simulink model "redocking_site"  (R2020b)
settings: Solver=FixedStepDiscrete  StartTime=0.0  StopTime=stopTime  FixedStep=2.0833333333333333e-05  RelTol=1e-3
values from neighbouring files (symbols this model uses):
  t_rd_init = t_rd_rest + 0.02e-3*spont - t_rd_jump    (= 0.0156)    [modelparameters.m]
  unitRateInterval = -log(randNums(k))/tdres    [SpikeGenerator_matt.m]    (also in modelparameters.m = 87745)
libraries: hdlsllib x1
settings Model: Creator=Ross  LastModifiedBy=tyler
settings SolverCC: AutoInsertRateTranBlk=on
settings DataIOCC: SaveOutput=off  SaveTime=off  ReturnWorkspaceOutputs=off
settings OptimizationCC: BlockReduction=off  ConditionallyExecuteInputs=off  DefaultParameterBehavior=Inlined
settings DebuggingCC: ReadBeforeWriteMsg=DisableAll  WriteAfterWriteMsg=DisableAll  WriteAfterReadMsg=DisableAll  AlgebraicLoopMsg=error  MultiTaskDSMMsg=none  SingleTaskRateTransMsg=error  PregeneratedLibrarySubsystemCodeDiagnostic=none  ArithmeticOperatorsInVariantConditions=warning
settings HardwareCC: ProdBitPerPointer=32  ProdBitPerSizeT=32  ProdBitPerPtrDiffT=32  ProdLargestAtomicFloat=None  ProdIntDivRoundTo=Undefined  ProdEndianess=Unspecified  ProdWordSize=32  ProdHWDeviceType=ASIC/FPGA->ASIC/FPGA  TargetBitPerPointer=64  TargetBitPerSizeT=64  TargetBitPerPtrDiffT=64  TargetLongLongMode=on  TargetIntDivRoundTo=Zero  TargetEndianess=LittleEndian  TargetWordSize=64  TargetHWDeviceType=Custom Processor->MATLAB Host Computer  ProdEqTarget=off
settings ModelReferenceCC: UpdateModelReferenceTargets=IfOutOfDate
settings SFSimCC: SFSimEcho=off  SimUseLocalCustomCode=off  CustomCodeUndefinedFunction=UseInterfaceOnly
settings RTWCC: RTWUseLocalCustomCode=off

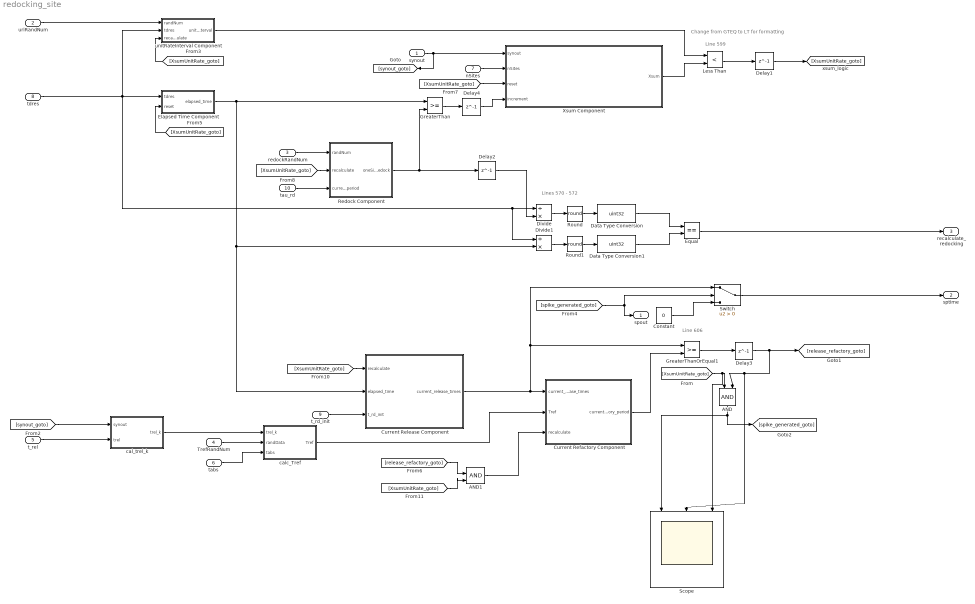
== system redocking_site ==
  note: Change from GTEQ to LT for formatting
  note: Line 606
  note: Lines 570 - 572
  note: Line 599
  synout : Inport  OutDataTypeStr=single  PortDimensions=1  SampleTime=[2.0833333333333333e-05,0]
  uriRandNum : Inport  Port=2  OutDataTypeStr=single  PortDimensions=1  SampleTime=[2.0833333333333333e-05,0]
  redockRandNum : Inport  Port=3  OutDataTypeStr=single  PortDimensions=1  SampleTime=[2.0833333333333333e-05,0]
  TrefRandNum : Inport  Port=4  OutDataTypeStr=single  PortDimensions=1  SampleTime=[2.0833333333333333e-05,0]
  t_rel : Inport  Port=5  OutDataTypeStr=single  PortDimensions=1  SampleTime=[2.0833333333333333e-05,0]
  tabs : Inport  Port=6  OutDataTypeStr=single  PortDimensions=1  SampleTime=[2.0833333333333333e-05,0]
  nSites : Inport  Port=7  OutDataTypeStr=single  PortDimensions=1  SampleTime=[2.0833333333333333e-05,0]
  tdres : Inport  Port=8  OutDataTypeStr=single  PortDimensions=1  SampleTime=[2.0833333333333333e-05,0]
  t_rd_init : Inport  Port=9  OutDataTypeStr=single  PortDimensions=1  SampleTime=[2.0833333333333333e-05,0]
  tau_rd : Inport  Port=10  OutDataTypeStr=single  PortDimensions=1  SampleTime=[2.0833333333333333e-05,0]
  AND : Logic  IconShape=distinctive  AllPortsSameDT=off  OutDataTypeStr=boolean
  AND1 : Logic  IconShape=distinctive  AllPortsSameDT=off  OutDataTypeStr=boolean
  Constant : Constant  Value=0  OutDataTypeStr=single  SampleTime=-1
  Current Refactory Component : Subsystem
  Current Release Component : Subsystem
  Data Type Conversion : DataTypeConversion  OutDataTypeStr=uint32
  Data Type Conversion1 : DataTypeConversion  OutDataTypeStr=uint32
  Delay{1..4} (4 alike) : Delay  DelayLength=1
  Divide : Product  Inputs=/*
  Divide1 : Product  Inputs=/*
  Elapsed Time Component : Subsystem
  Equal : RelationalOperator  Operator===  OutDataTypeStr=boolean  RndMeth=Simplest
  GreaterThan : RelationalOperator  OutDataTypeStr=boolean  RndMeth=Simplest
  GreaterThanOrEqual1 : RelationalOperator  OutDataTypeStr=boolean  RndMeth=Simplest
  Less Than : RelationalOperator  Operator=<  OutDataTypeStr=boolean  RndMeth=Simplest
  Redock Component : Subsystem
  Round : Rounding  Operator=round
  Round1 : Rounding  Operator=round
  Scope : Scope  NumInputPorts=3
  Switch : Switch  Criteria=u2 > Threshold
  Xsum Component : Subsystem
  cal_trel_k : Subsystem
  calc_Tref : Subsystem
  unitRateInterval Component : Subsystem
  spout : Outport  OutDataTypeStr=boolean  PortDimensions=1  SampleTime=[2.0833333333333333e-05,0]  InitialOutput=0
  sptime : Outport  Port=2  OutDataTypeStr=single  PortDimensions=1  SampleTime=[2.0833333333333333e-05,0]  InitialOutput=0
  recalculate_redocking : Outport  Port=3  OutDataTypeStr=boolean  PortDimensions=1  SampleTime=[2.0833333333333333e-05,0]
  wires:
  [spike_generated_goto] -> spout/1, Switch/2
  GreaterThanOrEqual1/1 -> Delay3/1
  Constant/1 -> Switch/3
  unitRateInterval Component/1(unitRateInterval) -> Less Than/1
  Xsum Component/1(Xsum) -> Less Than/2
  redockRandNum/1 -> Redock Component/1(randNum)
  [XsumUnitRate_goto] -> AND1/2
  [XsumUnitRate_goto] -> Elapsed Time Component/2(reset)
  [XsumUnitRate_goto] -> Xsum Component/3(reset)
  [XsumUnitRate_goto] -> unitRateInterval Component/3(recalculate)
  Delay2/1 -> Divide/2
  [XsumUnitRate_goto] -> Current Release Component/1(recalculate)
  calc_Tref/1(Tref) -> Current Refactory Component/2(Tref)
  [synout_goto] -> cal_trel_k/1(synout)
  uriRandNum/1 -> unitRateInterval Component/1(randNum)
  Delay1/1 -> [XsumUnitRate_goto]
  cal_trel_k/1(trel_k) -> calc_Tref/1(trel_k)
  t_rel/1 -> cal_trel_k/2(trel)
  Switch/1 -> sptime/1
  Equal/1 -> recalculate_redocking/1
  tabs/1 -> calc_Tref/3(tabs)
  Delay3/1 -> AND/2, Scope/2, [release_refactory_goto]
  Less Than/1 -> Delay1/1
  tdres/1 -> Divide1/1, Divide/1, unitRateInterval Component/2(tdres), Elapsed Time Component/1(tdres)
  Divide1/1 -> Round1/1
  [release_refactory_goto] -> AND1/1
  nSites/1 -> Xsum Component/2(nSites)
  [XsumUnitRate_goto] -> Redock Component/2(recalculate)
  Data Type Conversion1/1 -> Equal/2
  t_rd_init/1 -> Current Release Component/3(t_rd_init)
  TrefRandNum/1 -> calc_Tref/2(randData)
  Round/1 -> Data Type Conversion/1
  Round1/1 -> Data Type Conversion1/1
  tau_rd/1 -> Redock Component/3(current_redocking_period)
  synout/1 -> Xsum Component/1(synout), [synout_goto]
  AND/1 -> [spike_generated_goto], Scope/1
  [XsumUnitRate_goto] -> Scope/3, AND/1
  AND1/1 -> Current Refactory Component/3(recalculate)
  Divide/1 -> Round/1
  Data Type Conversion/1 -> Equal/1
  Current Refactory Component/1(current_refactory_period) -> GreaterThanOrEqual1/2
  Current Release Component/1(current_release_times) -> GreaterThanOrEqual1/1, Switch/1, Current Refactory Component/1(current_release_times)
  Elapsed Time Component/1(elapsed_time) -> GreaterThan/1, Current Release Component/2(elapsed_time), Divide1/2
  GreaterThan/1 -> Delay4/1
  Delay4/1 -> Xsum Component/4(increment)
  Redock Component/1(oneSiteRedock) -> GreaterThan/2, Delay2/1

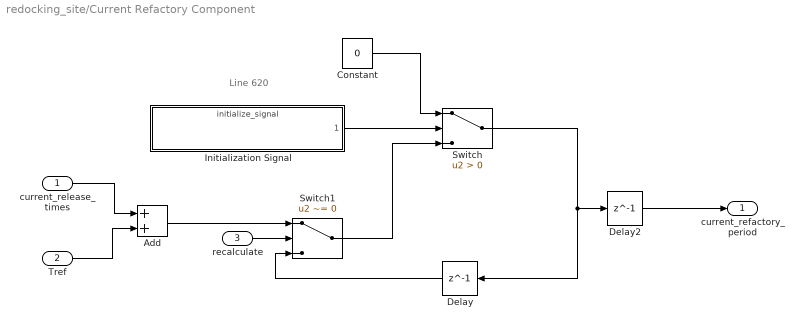
== system redocking_site/Current Refactory Component ==
  note: Line 620
  current_release_times : Inport
  Tref : Inport  Port=2
  recalculate : Inport  Port=3
  Add : Sum
  Constant : Constant  Value=0  OutDataTypeStr=single  SampleTime=-1
  Delay : Delay  DelayLength=1
  Delay2 : Delay  DelayLength=1
  Initialization Signal : ModelReference  ModelNameDialog=initialize_signal  SimulationMode=Normal  ModelReferenceVersion=1.282
  Switch : Switch  Criteria=u2 > Threshold  OutDataTypeStr=single
  Switch1 : Switch  Criteria=u2 ~= 0  OutDataTypeStr=single
  current_refactory_period : Outport
  wires:
  Delay/1 -> Switch1/3
  Switch/1 -> Delay2/1, Delay/1
  Switch1/1 -> Switch/3
  current_release_times/1 -> Add/1
  Tref/1 -> Add/2
  recalculate/1 -> Switch1/2
  Initialization Signal/1 -> Switch/2
  Constant/1 -> Switch/1
  Add/1 -> Switch1/1
  Delay2/1 -> current_refactory_period/1

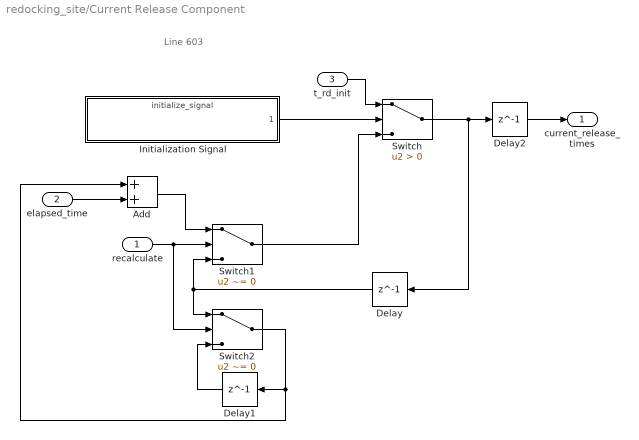
== system redocking_site/Current Release Component ==
  note: Line 603
  recalculate : Inport
  elapsed_time : Inport  Port=2
  t_rd_init : Inport  Port=3
  Add : Sum
  Delay : Delay  DelayLength=1
  Delay1 : Delay  DelayLength=1
  Delay2 : Delay  DelayLength=1
  Initialization Signal : ModelReference  ModelNameDialog=initialize_signal  SimulationMode=Normal  ModelReferenceVersion=1.282
  Switch : Switch  Criteria=u2 > Threshold  OutDataTypeStr=single
  Switch1 : Switch  Criteria=u2 ~= 0  OutDataTypeStr=single
  Switch2 : Switch  Criteria=u2 ~= 0  OutDataTypeStr=single
  current_release_times : Outport
  wires:
  Delay/1 -> Switch2/1, Switch1/3
  Switch/1 -> Delay2/1, Delay/1
  Switch1/1 -> Switch/3
  recalculate/1 -> Switch2/2, Switch1/2
  Add/1 -> Switch1/1
  Switch2/1 -> Add/1, Delay1/1
  elapsed_time/1 -> Add/2
  Initialization Signal/1 -> Switch/2
  t_rd_init/1 -> Switch/1
  Delay1/1 -> Switch2/3
  Delay2/1 -> current_release_times/1

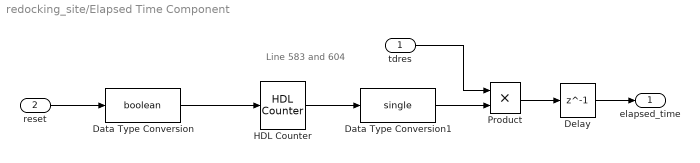
== system redocking_site/Elapsed Time Component ==
  note: Line 583 and 604
  tdres : Inport
  reset : Inport  Port=2
  Data Type Conversion : DataTypeConversion  OutDataTypeStr=boolean
  Data Type Conversion1 : DataTypeConversion  OutDataTypeStr=single
  Delay : Delay  DelayLength=1
  HDL Counter : hdlsllib/Sources/HDL Counter  CountType=Count limited  CountInit=0  CountStep=1  CountMax=1023  CountFromType=Initial value  CountFrom=0  CountResetPort=on  CountLoadPort=off  CountEnbPort=off  CountDirPort=off  CountDataType=Unsigned  CountWordLen=10  CountFracLen=0  CountSampTime=-1
  Product : Product  OutDataTypeStr=single
  elapsed_time : Outport
  wires:
  Data Type Conversion1/1 -> Product/2
  Data Type Conversion/1 -> HDL Counter/1
  Product/1 -> Delay/1
  tdres/1 -> Product/1
  HDL Counter/1 -> Data Type Conversion1/1
  reset/1 -> Data Type Conversion/1
  Delay/1 -> elapsed_time/1

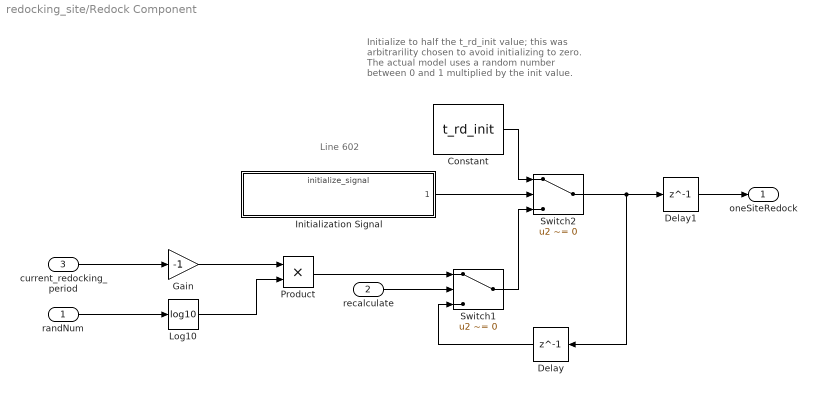
== system redocking_site/Redock Component ==
  note: Line 602
  note: Initialize to half the t_rd_init value; this was
      | arbitrarility chosen to avoid initializing to zero.
      | The actual model uses a random number
      | between 0 and 1 multiplied by the init value.
  randNum : Inport
  recalculate : Inport  Port=2
  current_redocking_period : Inport  Port=3
  Constant : Constant  Value=t_rd_init  OutDataTypeStr=single  SampleTime=-1
  Delay : Delay  DelayLength=1
  Delay1 : Delay  DelayLength=1
  Gain : Gain  Gain=-1
  Initialization Signal : ModelReference  ModelNameDialog=initialize_signal  SimulationMode=Normal  ModelReferenceVersion=1.282
  Log10 : Math  Operator=log10  SaturateOnIntegerOverflow=on
  Product : Product
  Switch1 : Switch  Criteria=u2 ~= 0  OutDataTypeStr=single
  Switch2 : Switch  Criteria=u2 ~= 0  OutDataTypeStr=single
  oneSiteRedock : Outport
  wires:
  Delay/1 -> Switch1/3
  Switch1/1 -> Switch2/3
  Initialization Signal/1 -> Switch2/2
  Constant/1 -> Switch2/1
  Switch2/1 -> Delay1/1, Delay/1
  Log10/1 -> Product/2
  Gain/1 -> Product/1
  current_redocking_period/1 -> Gain/1
  Product/1 -> Switch1/1
  randNum/1 -> Log10/1
  recalculate/1 -> Switch1/2
  Delay1/1 -> oneSiteRedock/1

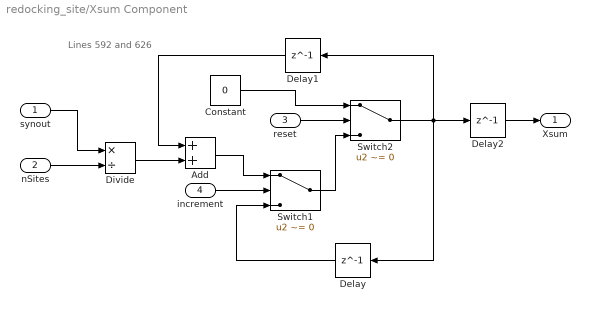
== system redocking_site/Xsum Component ==
  note: Lines 592 and 626
  synout : Inport
  nSites : Inport  Port=2
  reset : Inport  Port=3
  increment : Inport  Port=4
  Add : Sum
  Constant : Constant  Value=0  OutDataTypeStr=single  SampleTime=-1
  Delay : Delay  DelayLength=1
  Delay1 : Delay  DelayLength=1
  Delay2 : Delay  DelayLength=1
  Divide : Product  Inputs=*/
  Switch1 : Switch  Criteria=u2 ~= 0  OutDataTypeStr=single
  Switch2 : Switch  Criteria=u2 ~= 0  OutDataTypeStr=single
  Xsum : Outport
  wires:
  Delay1/1 -> Add/1
  Delay/1 -> Switch1/3
  Switch2/1 -> Delay2/1, Delay1/1, Delay/1
  Add/1 -> Switch1/1
  Divide/1 -> Add/2
  nSites/1 -> Divide/2
  synout/1 -> Divide/1
  Constant/1 -> Switch2/1
  Switch1/1 -> Switch2/3
  increment/1 -> Switch1/2
  reset/1 -> Switch2/2
  Delay2/1 -> Xsum/1

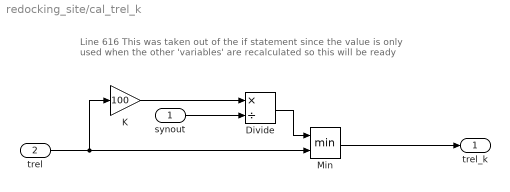
== system redocking_site/cal_trel_k ==
  note: Line 616
      | This was taken out of the if statement since the value is only used
      | when the other 'variables' are recalculated so this will be ready
  synout : Inport
  trel : Inport  Port=2
  Divide : Product  Inputs=*/
  K : Gain  Gain=100
  Min : MinMax  Inputs=2
  trel_k : Outport
  wires:
  trel/1 -> Min/2, K/1
  K/1 -> Divide/1
  Min/1 -> trel_k/1
  Divide/1 -> Min/1
  synout/1 -> Divide/2

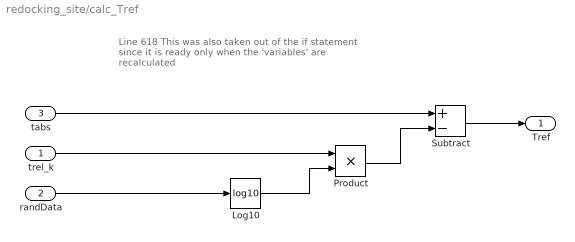
== system redocking_site/calc_Tref ==
  note: Line 618
      | This was also taken out of the if statement since
      | it is ready only when the 'variables' are recalculated
  trel_k : Inport
  randData : Inport  Port=2
  tabs : Inport  Port=3
  Log10 : Math  Operator=log10  SaturateOnIntegerOverflow=on
  Product : Product
  Subtract : Sum  Inputs=+-
  Tref : Outport
  wires:
  Subtract/1 -> Tref/1
  Product/1 -> Subtract/2
  Log10/1 -> Product/2
  trel_k/1 -> Product/1
  randData/1 -> Log10/1
  tabs/1 -> Subtract/1

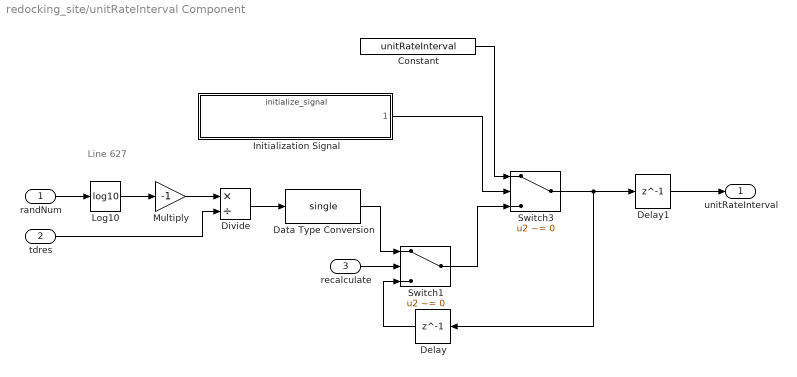
== system redocking_site/unitRateInterval Component ==
  note: Line 627
  randNum : Inport
  tdres : Inport  Port=2
  recalculate : Inport  Port=3
  Constant : Constant  Value=unitRateInterval  OutDataTypeStr=single  SampleTime=-1
  Data Type Conversion : DataTypeConversion  OutDataTypeStr=single
  Delay : Delay  DelayLength=1
  Delay1 : Delay  DelayLength=1
  Divide : Product  Inputs=*/
  Initialization Signal : ModelReference  ModelNameDialog=initialize_signal  SimulationMode=Normal  ModelReferenceVersion=1.282
  Log10 : Math  Operator=log10  SaturateOnIntegerOverflow=on
  Multiply : Gain  Gain=-1
  Switch1 : Switch  Criteria=u2 ~= 0  OutDataTypeStr=single
  Switch3 : Switch  Criteria=u2 ~= 0  OutDataTypeStr=single
  unitRateInterval : Outport
  wires:
  Delay/1 -> Switch1/3
  Switch1/1 -> Switch3/3
  recalculate/1 -> Switch1/2
  randNum/1 -> Log10/1
  Log10/1 -> Multiply/1
  Data Type Conversion/1 -> Switch1/1
  Divide/1 -> Data Type Conversion/1
  tdres/1 -> Divide/2
  Multiply/1 -> Divide/1
  Constant/1 -> Switch3/1
  Switch3/1 -> Delay/1, Delay1/1
  Initialization Signal/1 -> Switch3/2
  Delay1/1 -> unitRateInterval/1
